simulink model "ivedsp3"  (Simulink 7.6)
settings: Solver=FixedStepDiscrete  StartTime=0.0  StopTime=10  FixedStep=1  RelTol=1e-3
libraries: simulink x21
settings Model: Creator=jordan  LastModifiedBy=jordan
settings DataIOCC: LimitDataPoints=off  SaveOutput=off  SignalLogging=off  DSMLogging=off  SaveTime=off
settings OptimizationCC: BlockReduction=off  ConditionallyExecuteInputs=off  InlineParams=on

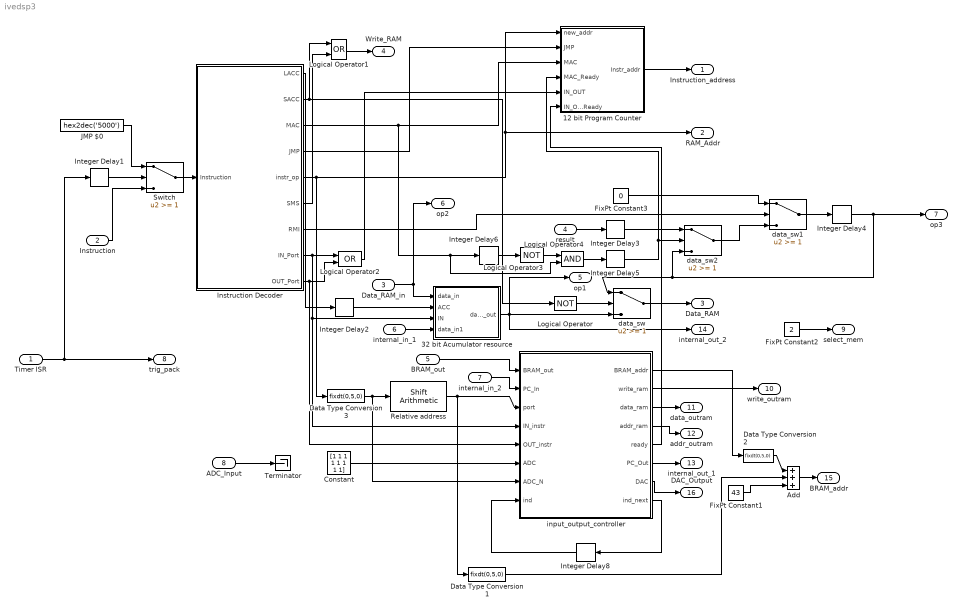
== system ivedsp3 ==
  Timer ISR : Inport  OutDataTypeStr=boolean
  Instruction : Inport  Port=2  OutDataTypeStr=uint16
  Data_RAM_in : Inport  Port=3  OutDataTypeStr=uint32
  result : Inport  Port=4  OutDataTypeStr=uint32
  BRAM_out : Inport  Port=5  OutDataTypeStr=uint8
  internal_in_1 : Inport  Port=6  OutDataTypeStr=uint32
  internal_in_2 : Inport  Port=7  OutDataTypeStr=uint8  PortDimensions=4
  ADC_Input : Inport  Port=8  OutDataTypeStr=uint8  PortDimensions=8
  12 bit Program Counter : Subsystem
  32 bit Acumulator resource : Subsystem
  Add : Sum  Inputs=+++  AccumDataTypeStr=fixdt(0,11,0)  OutDataTypeStr=fixdt(0,11,0)
  Constant : Constant  Value=[1 1 1 1 1 1 1 1]  OutDataTypeStr=uint8
  Data Type Conversion1 : DataTypeConversion  OutDataTypeStr=fixdt(0,5,0)  SaturateOnIntegerOverflow=on
  Data Type Conversion2 : DataTypeConversion  OutDataTypeStr=fixdt(0,5,0)
  Data Type Conversion3 : DataTypeConversion  OutDataTypeStr=fixdt(0,5,0)
  FixPt Constant1 : Constant  DisableCoverage=on  Value=43  OutDataTypeStr=fixdt(0,11,0)
  FixPt Constant2 : Constant  DisableCoverage=on  Value=2  OutDataTypeStr=fixdt(0,4,0)
  FixPt Constant3 : Constant  DisableCoverage=on  Value=0  OutDataTypeStr=uint32
  Instruction Decoder : Subsystem
  Integer Delay{1..4,6,8} (6 alike) : simulink/Discrete/Integer Delay  NumDelays=1  vinit=0.0  samptime=-1
  Integer Delay5 : simulink/Discrete/Integer Delay  NumDelays=3  vinit=0.0  samptime=-1
  JMP $0 : Constant  DisableCoverage=on  Value=hex2dec('5000')  OutDataTypeStr=Inherit: Inherit via back propagation
  Logical Operator : Logic  Operator=NOT  AllPortsSameDT=off  OutDataTypeStr=boolean
  Logical Operator1 : Logic  Operator=OR  AllPortsSameDT=off  OutDataTypeStr=boolean
  Logical Operator2 : Logic  Operator=OR  AllPortsSameDT=off  OutDataTypeStr=boolean
  Logical Operator3 : Logic  Operator=NOT  AllPortsSameDT=off  OutDataTypeStr=boolean
  Logical Operator4 : Logic  AllPortsSameDT=off  OutDataTypeStr=boolean
  Relative address : simulink/Logic and Bit Operations/Shift Arithmetic  SystemSampleTime=-1  nBitShiftRight=-2  nBinPtShiftRight=0
  Switch : Switch  Threshold=1
  Terminator : Terminator
  data_sw : Switch  Threshold=1
  data_sw1 : Switch  Threshold=1
  data_sw2 : Switch  Threshold=1
  input_output_controller : Stateflow chart  TreatAsAtomicUnit=on
  Instruction_address : Outport  OutDataTypeStr=fixdt(0,12,0)
  RAM_Addr : Outport  Port=2  OutDataTypeStr=fixdt(0,12,0)
  Data_RAM : Outport  Port=3  OutDataTypeStr=uint32
  Write_RAM : Outport  Port=4  OutDataTypeStr=boolean
  op1 : Outport  Port=5  OutDataTypeStr=uint32
  op2 : Outport  Port=6  OutDataTypeStr=uint32
  op3 : Outport  Port=7  OutDataTypeStr=uint32
  trig_pack : Outport  Port=8
  select_mem : Outport  Port=9
  write_outram : Outport  Port=10
  data_outram : Outport  Port=11
  addr_outram : Outport  Port=12
  internal_out_1 : Outport  Port=13
  internal_out_2 : Outport  Port=14  OutDataTypeStr=uint32
  BRAM_addr : Outport  Port=15
  DAC_Output : Outport  Port=16
  wires:
  32 bit Acumulator resource/1(data_out) -> data_sw/3, op1/1, internal_out_2/1
  Data_RAM_in/1 -> 32 bit Acumulator resource/1(data_in), op2/1
  Instruction Decoder/5(instr_op) -> 12 bit Program Counter/1(new_addr), RAM_Addr/1, Data Type Conversion3/1
  Instruction Decoder/1(LACC) -> Integer Delay2/1
  Integer Delay2/1 -> 32 bit Acumulator resource/2(ACC)
  Instruction Decoder/2(SACC) -> Logical Operator/1, Logical Operator1/1
  Logical Operator/1 -> data_sw/2
  Instruction Decoder/4(JMP) -> 12 bit Program Counter/2(JMP)
  Instruction Decoder/3(MAC) -> 12 bit Program Counter/3(MAC), Logical Operator4/2, Integer Delay6/1
  Instruction Decoder/7(RMI) -> data_sw1/2
  Instruction Decoder/6(SMS) -> Logical Operator1/2
  Instruction Decoder/8(IN_Port) -> 32 bit Acumulator resource/3(IN), input_output_controller/4(IN_instr), Logical Operator2/1
  Data Type Conversion3/1 -> Relative address/1, input_output_controller/7(ADC_N)
  Switch/1 -> Instruction Decoder/1(Instruction)
  JMP $0/1 -> Switch/1
  12 bit Program Counter/1(Instr_addr) -> Instruction_address/1
  Instruction/1 -> Switch/3
  data_sw/1 -> Data_RAM/1
  Logical Operator1/1 -> Write_RAM/1
  result/1 -> Integer Delay3/1
  Instruction Decoder/9(OUT_Port) -> Logical Operator2/2, input_output_controller/5(OUT_instr)
  BRAM_out/1 -> input_output_controller/1(BRAM_out)
  input_output_controller/4(addr_ram) -> addr_outram/1
  input_output_controller/2(write_ram) -> write_outram/1
  input_output_controller/3(data_ram) -> data_outram/1
  input_output_controller/1(BRAM_addr) -> Data Type Conversion2/1
  Relative address/1 -> Data Type Conversion1/1, input_output_controller/3(port)
  input_output_controller/5(ready) -> 12 bit Program Counter/6(IN_OUT_Ready)
  Logical Operator2/1 -> 12 bit Program Counter/5(IN_OUT)
  internal_in_1/1 -> 32 bit Acumulator resource/4(data_in1)
  internal_in_2/1 -> input_output_controller/2(PC_In)
  Integer Delay1/1 -> Switch/2
  input_output_controller/6(PC_Out) -> internal_out_1/1
  Add/1 -> BRAM_addr/1
  Data Type Conversion1/1 -> Add/2
  FixPt Constant1/1 -> Add/3
  FixPt Constant2/1 -> select_mem/1
  Timer ISR/1 -> trig_pack/1, Integer Delay1/1
  Data Type Conversion2/1 -> Add/1
  Integer Delay4/1 -> op3/1, data_sw2/3, data_sw/1
  data_sw1/1 -> Integer Delay4/1
  FixPt Constant3/1 -> data_sw1/1
  data_sw2/1 -> data_sw1/3
  Integer Delay3/1 -> data_sw2/1
  Integer Delay5/1 -> 12 bit Program Counter/4(MAC_Ready), data_sw2/2
  Integer Delay6/1 -> Logical Operator3/1
  Logical Operator3/1 -> Logical Operator4/1
  Logical Operator4/1 -> Integer Delay5/1
  ADC_Input/1 -> Terminator/1
  input_output_controller/7(DAC) -> DAC_Output/1
  Constant/1 -> input_output_controller/6(ADC)
  input_output_controller/8(ind_next) -> Integer Delay8/1
  Integer Delay8/1 -> input_output_controller/8(ind)

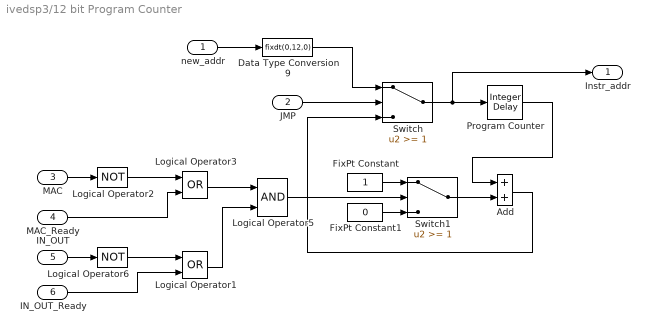
== system ivedsp3/12 bit Program Counter ==
  new_addr : Inport
  JMP : Inport  Port=2
  MAC : Inport  Port=3  OutDataTypeStr=boolean
  MAC_Ready : Inport  Port=4  OutDataTypeStr=boolean
  IN_OUT : Inport  Port=5  OutDataTypeStr=boolean
  IN_OUT_Ready : Inport  Port=6  OutDataTypeStr=boolean
  Add : Sum  AccumDataTypeStr=fixdt(0,12,0)  OutDataTypeStr=fixdt(0,12,0)
  Data Type Conversion9 : DataTypeConversion  OutDataTypeStr=fixdt(0,12,0)
  FixPt Constant : Constant  DisableCoverage=on  OutDataTypeStr=fixdt(0,12,0)
  FixPt Constant1 : Constant  DisableCoverage=on  Value=0  OutDataTypeStr=fixdt(0,12,0)
  Logical Operator1 : Logic  Operator=OR  AllPortsSameDT=off  OutDataTypeStr=boolean
  Logical Operator2 : Logic  Operator=NOT  AllPortsSameDT=off  OutDataTypeStr=boolean
  Logical Operator3 : Logic  Operator=OR  AllPortsSameDT=off  OutDataTypeStr=boolean
  Logical Operator5 : Logic  AllPortsSameDT=off  OutDataTypeStr=boolean
  Logical Operator6 : Logic  Operator=NOT  AllPortsSameDT=off  OutDataTypeStr=boolean
  Program Counter : simulink/Discrete/Integer Delay  NumDelays=1  vinit=0.0  samptime=-1
  Switch : Switch  Threshold=1
  Switch1 : Switch  Threshold=1
  Instr_addr : Outport  InitialOutput=0
  wires:
  JMP/1 -> Switch/2
  new_addr/1 -> Data Type Conversion9/1
  Program Counter/1 -> Add/1
  Switch/1 -> Program Counter/1, Instr_addr/1
  FixPt Constant/1 -> Switch1/1
  Add/1 -> Switch/3
  Data Type Conversion9/1 -> Switch/1
  Switch1/1 -> Add/2
  FixPt Constant1/1 -> Switch1/3
  Logical Operator3/1 -> Logical Operator5/1
  Logical Operator2/1 -> Logical Operator3/1
  MAC/1 -> Logical Operator2/1
  Logical Operator1/1 -> Logical Operator5/2
  Logical Operator6/1 -> Logical Operator1/1
  IN_OUT/1 -> Logical Operator6/1
  IN_OUT_Ready/1 -> Logical Operator1/2
  Logical Operator5/1 -> Switch1/2
  MAC_Ready/1 -> Logical Operator3/2

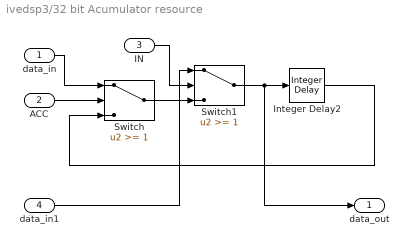
== system ivedsp3/32 bit Acumulator resource ==
  data_in : Inport
  ACC : Inport  Port=2
  IN : Inport  Port=3
  data_in1 : Inport  Port=4
  Integer Delay2 : simulink/Discrete/Integer Delay  NumDelays=1  vinit=0.0  samptime=-1
  Switch : Switch  Threshold=1
  Switch1 : Switch  Threshold=1
  data_out : Outport  OutDataTypeStr=uint32
  wires:
  Switch/1 -> Switch1/3
  Integer Delay2/1 -> Switch/3
  data_in/1 -> Switch/1
  ACC/1 -> Switch/2
  Switch1/1 -> Integer Delay2/1, data_out/1
  IN/1 -> Switch1/2
  data_in1/1 -> Switch1/1

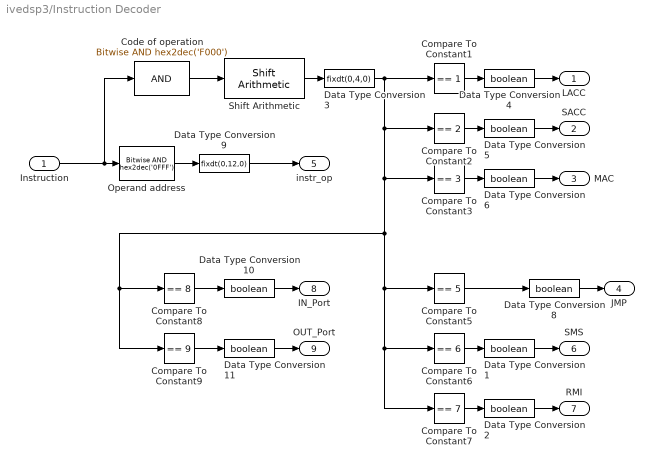
== system ivedsp3/Instruction Decoder ==
  Instruction : Inport  OutDataTypeStr=uint16
  Code of operation : simulink/Logic and Bit Operations/Bitwise Operator  logicop=AND  UseBitMask=on  BitMask=hex2dec('F000')  BitMaskRealWorld=Stored Integer
  Compare To Constant1 : simulink/Logic and Bit Operations/Compare To Constant  SystemSampleTime=-1  relop===  const=1  LogicOutDataTypeMode=boolean
  Compare To Constant2 : simulink/Logic and Bit Operations/Compare To Constant  SystemSampleTime=-1  relop===  const=2  LogicOutDataTypeMode=boolean
  Compare To Constant3 : simulink/Logic and Bit Operations/Compare To Constant  SystemSampleTime=-1  relop===  const=3  LogicOutDataTypeMode=boolean
  Compare To Constant5 : simulink/Logic and Bit Operations/Compare To Constant  SystemSampleTime=-1  relop===  const=5  LogicOutDataTypeMode=boolean
  Compare To Constant6 : simulink/Logic and Bit Operations/Compare To Constant  SystemSampleTime=-1  relop===  const=6  LogicOutDataTypeMode=boolean
  Compare To Constant7 : simulink/Logic and Bit Operations/Compare To Constant  SystemSampleTime=-1  relop===  const=7  LogicOutDataTypeMode=boolean
  Compare To Constant8 : simulink/Logic and Bit Operations/Compare To Constant  SystemSampleTime=-1  relop===  const=8  LogicOutDataTypeMode=boolean
  Compare To Constant9 : simulink/Logic and Bit Operations/Compare To Constant  SystemSampleTime=-1  relop===  const=9  LogicOutDataTypeMode=boolean
  Data Type Conversion{1..2,4..6,8,10..11} (8 alike) : DataTypeConversion  OutDataTypeStr=boolean
  Data Type Conversion3 : DataTypeConversion  OutDataTypeStr=fixdt(0,4,0)
  Data Type Conversion9 : DataTypeConversion  OutDataTypeStr=fixdt(0,12,0)
  Operand address : simulink/Logic and Bit Operations/Bitwise Operator  logicop=AND  UseBitMask=on  BitMask=hex2dec('0FFF')  BitMaskRealWorld=Stored Integer
  Shift Arithmetic : simulink/Logic and Bit Operations/Shift Arithmetic  SystemSampleTime=-1  nBitShiftRight=12  nBinPtShiftRight=0
  LACC : Outport
  SACC : Outport  Port=2
  MAC : Outport  Port=3
  JMP : Outport  Port=4
  instr_op : Outport  Port=5
  SMS : Outport  Port=6
  RMI : Outport  Port=7
  IN_Port : Outport  Port=8
  OUT_Port : Outport  Port=9
  wires:
  Instruction/1 -> Operand address/1, Code of operation/1
  Code of operation/1 -> Shift Arithmetic/1
  Shift Arithmetic/1 -> Data Type Conversion3/1
  Data Type Conversion3/1 -> Compare To Constant6/1, Compare To Constant7/1, Compare To Constant5/1, Compare To Constant8/1, Compare To Constant9/1, Compare To Constant3/1, Compare To Constant2/1, Compare To Constant1/1
  Compare To Constant1/1 -> Data Type Conversion4/1
  Compare To Constant2/1 -> Data Type Conversion5/1
  Compare To Constant3/1 -> Data Type Conversion6/1
  Compare To Constant5/1 -> Data Type Conversion8/1
  Operand address/1 -> Data Type Conversion9/1
  Data Type Conversion4/1 -> LACC/1
  Data Type Conversion5/1 -> SACC/1
  Data Type Conversion9/1 -> instr_op/1
  Data Type Conversion6/1 -> MAC/1
  Data Type Conversion8/1 -> JMP/1
  Compare To Constant6/1 -> Data Type Conversion1/1
  Data Type Conversion1/1 -> SMS/1
  Compare To Constant7/1 -> Data Type Conversion2/1
  Data Type Conversion2/1 -> RMI/1
  Compare To Constant8/1 -> Data Type Conversion10/1
  Data Type Conversion10/1 -> IN_Port/1
  Compare To Constant9/1 -> Data Type Conversion11/1
  Data Type Conversion11/1 -> OUT_Port/1

== stateflow chart input_output_controller ==
  settings: executeAtInitialization=1
  state IN_Wait
  state Receive
  state OUT_Wait
  state IN_Wait2
  state IN_Wait3
  state Wait
  state Wait4
  state IN_Wait10
  state IN_Wait4
  state IN_Wait1
  state IN_Wait5
  state IN_Wait6
  state IN_Wait7
  state IN_Wait8
  state IN_Wait9
  state ADC
  state Ready
  state DAC
  IN_Wait5 -> IN_Wait : {PC_Out[0]=BRAM_out;
      | BRAM_addr=1;}
  IN_Wait8 -> IN_Wait9 : {PC_Out[3]=BRAM_out;}
  Wait4 -> IN_Wait10 : {ready=0;}
  (junction 21) -> Wait4 [order 1] : [ind==4]{
      | write_ram=0;
      | ready=1;}
  IN_Wait7 -> IN_Wait4 : {PC_Out[2]=BRAM_out;
      | BRAM_addr=3;}
  Receive -> Wait [order 1] : [OUT_instr==1]{
      | ready=0;}
  IN_Wait6 -> IN_Wait3 : {PC_Out[1]=BRAM_out;
      | BRAM_addr=2;}
  (junction 21) -> OUT_Wait [order 2] : {addr_ram=addr_ram+1;
      | data_ram=PC_In[ind];
      | ind_next=ind+1;}
  OUT_Wait -> (junction 21)
  (junction 30) -> (junction 31) [order 1] : [ADC_N>=10]
  (junction 22) -> IN_Wait1 [order 2] : {BRAM_addr=0;}
  (junction 30) -> OUT_Wait [order 2] : {addr_ram=port;
      | write_ram=1;
      | data_ram=PC_In[0];
      | ind_next=0;}
  (default) -> Receive
  Receive -> IN_Wait2 [order 2] : [IN_instr==1]{ready=0;}
  IN_Wait1 -> IN_Wait5
  IN_Wait -> IN_Wait6
  IN_Wait3 -> IN_Wait7
  IN_Wait4 -> IN_Wait8
  IN_Wait9 -> Wait4 : {ready=1;}
  IN_Wait2 -> (junction 22)
  (junction 22) -> ADC [order 1] : [ADC_N>=10]
  ADC -> (junction 23)
  (junction 23) -> (junction 24) [order 1] : [ADC_N==10]{
      | PC_Out[0]=ADC[0];
      | PC_Out[1]=ADC[1];
      | PC_Out[2]=ADC[2];
      | PC_Out[3]=ADC[3];}
  (junction 23) -> (junction 25) [order 2] : [ADC_N==11]{
      | PC_Out[0]=ADC[4];
      | PC_Out[1]=ADC[5];
      | PC_Out[2]=ADC[6];
      | PC_Out[3]=ADC[7];}
  (junction 24) -> (junction 25)
  (junction 25) -> Ready
  (junction 26) -> Wait4 : {ready=1;}
  (junction 31) -> DAC
  IN_Wait10 -> Receive
  DAC -> (junction 27)
  (junction 27) -> (junction 28) [order 1] : [ADC_N==10]{
      | DAC[0]=PC_In[0];
      | DAC[1]=PC_In[1];
      | DAC[2]=PC_In[2];
      | DAC[3]=PC_In[3];}
  (junction 27) -> (junction 29) [order 2] : [ADC_N==11]{
      | DAC[4]=PC_In[0];
      | DAC[5]=PC_In[1];
      | DAC[6]=PC_In[2];
      | DAC[7]=PC_In[3];}
  (junction 28) -> (junction 29)
  (junction 29) -> (junction 26)
  Ready -> IN_Wait9
  Wait -> (junction 30)
  data: BRAM_out input uint8; BRAM_addr output fixdt(0,2,0) =0; write_ram output boolean =0; data_ram output uint8; addr_ram output fixdt(0,14,0) =0; PC_In input uint8 size=4; port input fixdt(0,5,0); IN_instr input boolean; ready output boolean; OUT_instr input boolean; PC_Out output uint8 size=4; ADC input uint8 size=8; ADC_N input fixdt(0,5,0); DAC output uint8 size=8; ind_next output fixdt(0,5,0) =0; ind input fixdt(0,5,0)
